simulink library "lib_dsphdlutils_v1"  (R2019b)
settings: Solver=ode45  StartTime=0.0  StopTime=10.0  RelTol=1e-3  EnableMultiTasking=on
libraries: simulink x4, dspstat3 x1, dspmathops x1
settings Model: Creator=mbabst  LastModifiedBy=mbabst
settings DataIOCC: LimitDataPoints=on
settings OptimizationCC: LifeSpan=inf
settings DebuggingCC: AllowSymbolicDim=off  SFUnexpectedBacktrackingDiag=warning  SFNoUnconditionalDefaultTransitionDiag=warning  SFExecutionAtInitializationDiag=none  ArithmeticOperatorsInVariantConditions=warning
settings SFSimCC: SimUseLocalCustomCode=off  CustomCodeUndefinedFunction=UseInterfaceOnly
settings RTWCC: RTWUseLocalCustomCode=off
settings CodeAppCC: StateflowObjectComments=on
settings GRTTargetCC: TargetLangStandard=C89/C90 (ANSI)  GeneratePreprocessorConditionals=Disable all
settings ConfigComp: CovMetricSettings=dw  CovHtmlReporting=on  CovSaveCumulativeToWorkspaceVar=on  CovSaveSingleToWorkspaceVar=on  CovExternalEMLEnable=off

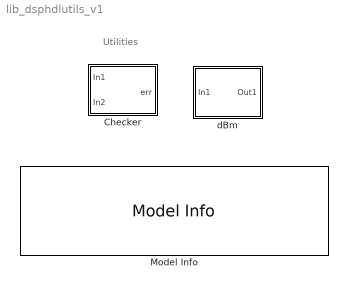
== system lib_dsphdlutils_v1 ==
  note: Utilities
  Checker : Subsystem  mask(Compare two signals){StopSim=on}
      mask prompts: StopSim "Stop Sim on Error"
      mask help:
      | Compare two signals and output the error.
      | If selected, the simulation can be stopped if there is a mismatch.
      mask init:
      | set_param([gcb '/Assertion' ], 'StopWhenAssertionFail', StopSim);
      | set_param([gcb '/Assertion' ], 'Enabled', StopSim);
      mask Display:
      | if StopSim
      |     disp('Compare\n(halt)');
      | else
      |     disp('Compare');
      | end
  Model Info : simulink/Model-Wide Utilities/Model Info  Frame=on  DisplayStringWithTags=|  HorizontalTextAlignment=Left  LeftAlignmentValue=0.02
      | Copyright (c) 2005-2021 DSPlogic, Inc.
      | Distributed under the terms of the Simplified BSD License.
      | The full license is in the file LICENSE, distributed with this software.
      | 
      | Model: %<ModelName> (v%<ModelVersion>)
      | Author: Michael Babst <mike.babst@dsplogic.com>
      | Created: by %<Creator> on %<Created>
      | Modified: by %<ModifiedBy> on %<LastModificationDate>
  dBm : Subsystem  mask(Signal level (dB)){units=dB, rohms=1}
      mask prompts: rohms "Reference Load (ohms)"
      mask help: This block computes the running average signal level in decibels.
      mask init:
      | switch units
      |     case 1
      |         dispstr = ['dB\n(' num2str(rohms) ' ohm)'];
      |         set_param([gcb '/dBconvert'], 'dBtype', 'dB');
      |     case 2
      |         dispstr = ['dBm\n(' num2str(rohms) ' ohm)'];
      |         set_param([gcb '/dBconvert'], 'dBtype', 'dBm');
      | end
      settings: PermitHierarchicalResolution=None
      mask TypeOptions units: dB | dBm
      mask Display: disp(dispstr);

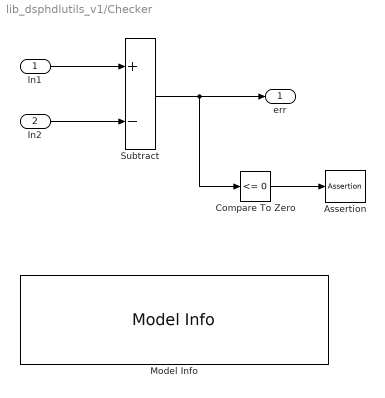
== system lib_dsphdlutils_v1/Checker ==
  In1 : Inport
  In2 : Inport  Port=2
  Assertion : Assertion
      settings: AttributesFormatString=|
      | %<BlockType>
      | %<StopWhenAssertionFail>
  Compare To Zero : simulink/Logic and Bit Operations/Compare To Zero  relop=<=  OutDataTypeStr=boolean
  Model Info : simulink/Model-Wide Utilities/Model Info  Frame=on  DisplayStringWithTags=|  HorizontalTextAlignment=Left  LeftAlignmentValue=0.02
      | Copyright (c) 2005-2021 DSPlogic, Inc.
      | Distributed under the terms of the Simplified BSD License.
      | The full license is in the file LICENSE, distributed with this software.
      | 
      | Model: %<ModelName> (v%<ModelVersion>)
      | Author: Michael Babst <mike.babst@dsplogic.com>
      | Created: by %<Creator> on %<Created>
      | Modified: by %<ModifiedBy> on %<LastModificationDate>
  Subtract : Sum  Inputs=+-
  err : Outport
  wires:
  Compare To Zero/1 -> Assertion/1
  In1/1 -> Subtract/1
  In2/1 -> Subtract/2
  Subtract/1 -> Compare To Zero/1, err/1

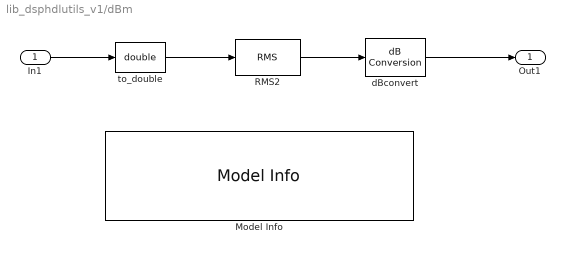
== system lib_dsphdlutils_v1/dBm ==
  In1 : Inport
  Model Info : simulink/Model-Wide Utilities/Model Info  Frame=on  DisplayStringWithTags=|  HorizontalTextAlignment=Left  LeftAlignmentValue=0.02
      | Copyright (c) 2005-2021 DSPlogic, Inc.
      | Distributed under the terms of the Simplified BSD License.
      | The full license is in the file LICENSE, distributed with this software.
      | 
      | Model: %<ModelName> (v%<ModelVersion>)
      | Author: Michael Babst <mike.babst@dsplogic.com>
      | Created: by %<Creator> on %<Created>
      | Modified: by %<ModifiedBy> on %<LastModificationDate>
  RMS2 : dspstat3/RMS  run=on  directionMode=Each column  dimension=1  reset_popup=None
  dBconvert : dspmathops/dB Conversion  dBtype=dB  intype=Amplitude  R=rohms  fuzz=off
      settings: SourceProductName=DSP System Toolbox
  to_double : DataTypeConversion  OutDataTypeStr=double
  Out1 : Outport
  wires:
  In1/1 -> to_double/1
  dBconvert/1 -> Out1/1
  RMS2/1 -> dBconvert/1
  to_double/1 -> RMS2/1
